simulink model "BLOC_Command"  (R2016a)
settings: Solver=VariableStepAuto  StartTime=0.0  StopTime=10.0  RelTol=1e-3
undefined symbols (not defined in the file): cmd_equivalent_conso_coef, cmd_qmax, cmd_specific_volume_l_per_g, fa_differential_ratio, fa_gearbox_efficiency, fa_gearbox_ratio, hev_dt, pla_wheel_radius, ra_differential_ratio, ra_transmission_efficiency
libraries: simulink x7
settings Model: Creator=Florent  LastModifiedBy=Florent
settings OptimizationCC: DefaultParameterBehavior=Inlined  OptimizeModelRefInitCode=on  LifeSpan=1
settings RTWCC: SystemTargetFile=ert.tlc  TemplateMakefile=ert_default_tmf  GenerateReport=on  IncludeHyperlinkInReport=on  LaunchReport=on  TargetLang=C++  GenerateTraceInfo=on  GenerateTraceReport=on  GenerateTraceReportSl=on  GenerateTraceReportSf=on  GenerateTraceReportEml=on
settings CodeAppCC: ForceParamTrailComments=on  OperatorAnnotations=on  SimulinkDataObjDesc=on  SFDataObjDesc=on  MATLABFcnDesc=on  InsertBlockDesc=on  MATLABSourceComments=on
settings ERTTargetCC: GenerateSampleERTMain=on  MultiInstanceERTCode=on  CodeInterfacePackaging=C++ class  InlinedParameterPlacement=NonHierarchical  RootIOFormat=Structure reference  ERTCustomFileTemplate=example_file_process.tlc

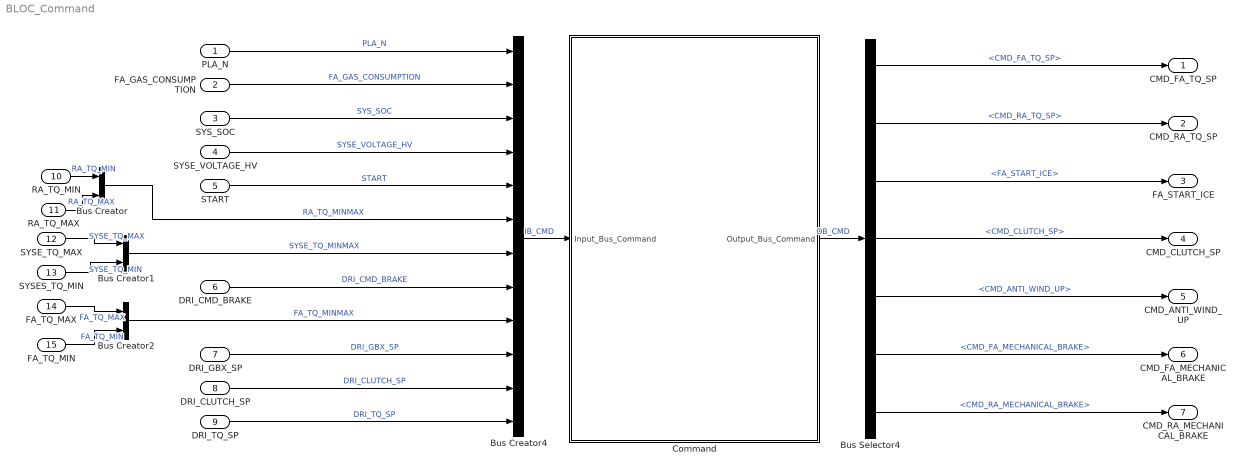
== system BLOC_Command ==
  PLA_N : Inport
  FA_GAS_CONSUMPTION : Inport  Port=2
  SYS_SOC : Inport  Port=3
  SYSE_VOLTAGE_HV : Inport  Port=4
  START : Inport  Port=5
  DRI_CMD_BRAKE : Inport  Port=6
  DRI_GBX_SP : Inport  Port=7
  DRI_CLUTCH_SP : Inport  Port=8
  DRI_TQ_SP : Inport  Port=9
  RA_TQ_MIN : Inport  Port=10
  RA_TQ_MAX : Inport  Port=11
  SYSE_TQ_MAX : Inport  Port=12
  SYSES_TQ_MIN : Inport  Port=13
  FA_TQ_MAX : Inport  Port=14
  FA_TQ_MIN : Inport  Port=15
  Bus Creator : BusCreator  Inputs=2
  Bus Creator1 : BusCreator  Inputs=2
  Bus Creator2 : BusCreator  Inputs=2
  Bus Creator4 : BusCreator  Inputs=12
  Bus Selector4 : BusSelector  OutputSignals=CMD_FA_TQ_SP,CMD_RA_TQ_SP,FA_START_ICE,CMD_CLUTCH_SP,CMD_ANTI_WIND_UP,CMD_FA_MECHANICAL_BRAKE,CMD_RA_MECHANICAL_BRAKE
  Command : Subsystem  TreatAsAtomicUnit=on
  CMD_FA_TQ_SP : Outport
  CMD_RA_TQ_SP : Outport  Port=2
  FA_START_ICE : Outport  Port=3
  CMD_CLUTCH_SP : Outport  Port=4
  CMD_ANTI_WIND_UP : Outport  Port=5
  CMD_FA_MECHANICAL_BRAKE : Outport  Port=6
  CMD_RA_MECHANICAL_BRAKE : Outport  Port=7
  wires:
  PLA_N/1 -> Bus Creator4/1  "PLA_N"
  FA_GAS_CONSUMPTION/1 -> Bus Creator4/2  "FA_GAS_CONSUMPTION"
  SYS_SOC/1 -> Bus Creator4/3  "SYS_SOC"
  SYSE_VOLTAGE_HV/1 -> Bus Creator4/4  "SYSE_VOLTAGE_HV"
  START/1 -> Bus Creator4/5  "START"
  Bus Creator/1 -> Bus Creator4/6  "RA_TQ_MINMAX"
  Bus Creator1/1 -> Bus Creator4/7  "SYSE_TQ_MINMAX"
  DRI_CMD_BRAKE/1 -> Bus Creator4/8  "DRI_CMD_BRAKE"
  Bus Creator2/1 -> Bus Creator4/9  "FA_TQ_MINMAX"
  DRI_GBX_SP/1 -> Bus Creator4/10  "DRI_GBX_SP"
  DRI_CLUTCH_SP/1 -> Bus Creator4/11  "DRI_CLUTCH_SP"
  DRI_TQ_SP/1 -> Bus Creator4/12  "DRI_TQ_SP"
  Bus Creator4/1 -> Command/1(Input_Bus_Command)  "IB_CMD"
  Command/1(Output_Bus_Command) -> Bus Selector4/1  "OB_CMD"
  Bus Selector4/1 -> CMD_FA_TQ_SP/1  "<CMD_FA_TQ_SP>"
  Bus Selector4/2 -> CMD_RA_TQ_SP/1  "<CMD_RA_TQ_SP>"
  Bus Selector4/3 -> FA_START_ICE/1  "<FA_START_ICE>"
  Bus Selector4/4 -> CMD_CLUTCH_SP/1  "<CMD_CLUTCH_SP>"
  Bus Selector4/5 -> CMD_ANTI_WIND_UP/1  "<CMD_ANTI_WIND_UP>"
  Bus Selector4/6 -> CMD_FA_MECHANICAL_BRAKE/1  "<CMD_FA_MECHANICAL_BRAKE>"
  Bus Selector4/7 -> CMD_RA_MECHANICAL_BRAKE/1  "<CMD_RA_MECHANICAL_BRAKE>"
  RA_TQ_MIN/1 -> Bus Creator/1  "RA_TQ_MIN"
  RA_TQ_MAX/1 -> Bus Creator/2  "RA_TQ_MAX"
  SYSE_TQ_MAX/1 -> Bus Creator1/1  "SYSE_TQ_MAX"
  SYSES_TQ_MIN/1 -> Bus Creator1/2  "SYSE_TQ_MIN"
  FA_TQ_MAX/1 -> Bus Creator2/1  "FA_TQ_MAX"
  FA_TQ_MIN/1 -> Bus Creator2/2  "FA_TQ_MIN"

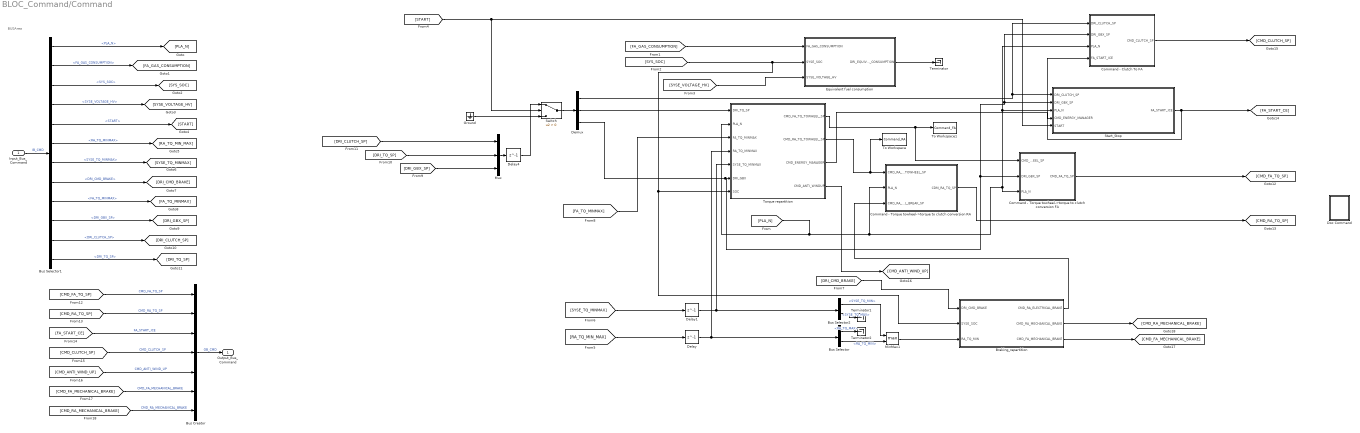
== system BLOC_Command/Command ==
  note: BUSArea
  Input_Bus_Command : Inport
  Braking_repartition : Subsystem
  Bus Creator : BusCreator  Inputs=7
  Bus Selector : BusSelector  OutputSignals=RA_TQ_MAX,RA_TQ_MIN
  Bus Selector1 : BusSelector  OutputSignals=PLA_N,FA_GAS_CONSUMPTION,SYS_SOC,SYSE_VOLTAGE_HV,START,RA_TQ_MINMAX,SYSE_TQ_MINMAX,DRI_CMD_BRAKE,FA_TQ_MINMAX,DRI_GBX_SP,DRI_CLUTCH_SP,DRI_TQ_SP
  Bus Selector2 : BusSelector  OutputSignals=SYSE_TQ_MIN,SYSE_TQ_MAX
  Command - Clutch To FA : Subsystem
  Command - Torque towheel->torque to clutch conversion FA : Subsystem
  Command - Torque towheel->torque to clutch conversion RA : Subsystem
  Delay : Delay  DelayLength=1
  Delay1 : Delay  DelayLength=1
  Delay4 : Delay  DelayLength=1  InitialCondition=1e-6
  Demux : Demux  Outputs=3
  Doc Command : Subsystem
      settings: OpenFcn=open('Documents\Command.pdf')
      mask Display: fprintf('DOC')
  Equivalent fuel consumption : Subsystem
  Ground : Ground
  MinMax1 : MinMax  Function=max  Inputs=2  SampleTime=hev_dt
  Mux : Mux  Inputs=3
  Start_Stop : Subsystem
  Switch : Switch  Criteria=u2 > Threshold
  Terminator : Terminator
  Terminator1 : Terminator
  Terminator2 : Terminator
  To Workspace : ToWorkspace  VariableName=Command_RA  SampleTime=-1
  To Workspace1 : ToWorkspace  VariableName=Command_FA  SampleTime=-1
  Torque repartition : Subsystem
  Output_Bus_Command : Outport
  wires:
  [FA_GAS_CONSUMPTION] -> Equivalent fuel consumption/1(FA_GAS_CONSUMPTION)
  [SYS_SOC] -> Equivalent fuel consumption/2(SYSE_SOC), Braking_repartition/2(SYSE_SOC), Torque repartition/7(SOC)
  [SYSE_VOLTAGE_HV] -> Equivalent fuel consumption/3(SYSE_VOLTAGE_HV)
  Torque repartition/1(CMD_FA_TQ_TOWHEEL_SP) -> To Workspace1/1, Command - Torque towheel->torque to clutch conversion FA/1(CMD_FA_TQ_TOWHEEL_SP)
  Equivalent fuel consumption/1(DRI_EQUIV_GAZ_CONSUMPTION) -> Terminator/1
  Command - Torque towheel->torque to clutch conversion FA/1(CMD_FA_TQ_SP) -> [CMD_FA_TQ_SP]
  [RA_TQ_MIN_MAX] -> Delay/1
  [SYSE_TQ_MINMAX] -> Delay1/1
  Bus Selector2/1 -> MinMax1/1  "<SYSE_TQ_MIN>"
  Bus Selector/2 -> MinMax1/2  "<RA_TQ_MIN>"
  Bus Selector/1 -> Terminator2/1  "<RA_TQ_MAX>"
  Bus Selector2/2 -> Terminator1/1  "<SYSE_TQ_MAX>"
  Command - Torque towheel->torque to clutch conversion RA/1(CDM_RA_TQ_SP) -> [CMD_RA_TQ_SP]
  Torque repartition/2(CMD_RA_TQ_TOWHEEL_SP) -> To Workspace/1, Command - Torque towheel->torque to clutch conversion RA/1(CMD_RA_TQ_TOWHEEL_SP)
  [START] -> Switch/2, Start_Stop/5(START)
  Start_Stop/1(FA_START_ICE) -> [FA_START_CE], Command - Clutch To FA/4(FA_START_ICE)
  [DRI_CMD_BRAKE] -> Braking_repartition/1(DRI_CMD_BRAKE)
  MinMax1/1 -> Braking_repartition/3(RA_TQ_MIN)
  [FA_TQ_MINMAX] -> Torque repartition/3(FA_TQ_MINMAX)
  Delay/1 -> Bus Selector/1, Torque repartition/4(RA_TQ_MINMAX)
  Delay1/1 -> Bus Selector2/1, Torque repartition/5(SYSE_TQ_MINMAX)
  Demux/1 -> Command - Clutch To FA/1(DRI_CLUTCH_SP), Start_Stop/1(DRI_CLUTCH_SP)
  [PLA_N] -> Command - Clutch To FA/3(PLA_N), Start_Stop/3(PLA_N), Command - Torque towheel->torque to clutch conversion FA/3(PLA_N), Command - Torque towheel->torque to clutch conversion RA/2(PLA_N), Torque repartition/2(PLA_N)
  Command - Clutch To FA/1("CMD_CLUTCH_SP ") -> [CMD_CLUTCH_SP]
  Torque repartition/3(CMD_ENERGY_MANAGER) -> Start_Stop/4(CMD_ENERGY_MANAGER)
  Torque repartition/4(CMD_ANTI_WINDUP) -> [CMD_ANTI_WIND_UP]
  Switch/1 -> Demux/1
  [DRI_GBX_SP] -> Mux/3
  Mux/1 -> Delay4/1
  Demux/3 -> Command - Clutch To FA/2(DRI_GBX_SP), Start_Stop/2(DRI_GBX_SP), Command - Torque towheel->torque to clutch conversion FA/2(DRI_GBX_SP), Torque repartition/6(DRI_GBX)
  Delay4/1 -> Switch/1
  Ground/1 -> Switch/3
  [DRI_CLUTCH_SP] -> Mux/1
  [DRI_TQ_SP] -> Mux/2
  Demux/2 -> Torque repartition/1(DRI_TQ_SP)
  Braking_repartition/1(CMD_RA_ELECTRICAL_BRAKE) -> Command - Torque towheel->torque to clutch conversion RA/3(CMD_RA_TQ_TOWHEEL_BREAK_SP)
  Braking_repartition/3(CMD_FA_MECHANICAL_BRAKE) -> [CMD_FA_MECHANICAL_BRAKE]
  Braking_repartition/2(CMD_RA_MECHANICAL_BRAKE) -> [CMD_RA_MECHANICAL_BRAKE]
  Input_Bus_Command/1 -> Bus Selector1/1  "IB_CMD"
  Bus Selector1/1 -> [PLA_N]  "<PLA_N>"
  Bus Selector1/2 -> [FA_GAS_CONSUMPTION]  "<FA_GAS_CONSUMPTION>"
  Bus Selector1/3 -> [SYS_SOC]  "<SYS_SOC>"
  Bus Selector1/4 -> [SYSE_VOLTAGE_HV]  "<SYSE_VOLTAGE_HV>"
  Bus Selector1/5 -> [START]  "<START>"
  Bus Selector1/6 -> [RA_TQ_MIN_MAX]  "<RA_TQ_MINMAX>"
  Bus Selector1/7 -> [SYSE_TQ_MINMAX]  "<SYSE_TQ_MINMAX>"
  Bus Selector1/8 -> [DRI_CMD_BRAKE]  "<DRI_CMD_BRAKE>"
  Bus Selector1/9 -> [FA_TQ_MINMAX]  "<FA_TQ_MINMAX>"
  Bus Selector1/10 -> [DRI_GBX_SP]  "<DRI_GBX_SP>"
  Bus Selector1/11 -> [DRI_CLUTCH_SP]  "<DRI_CLUTCH_SP>"
  Bus Selector1/12 -> [DRI_TQ_SP]  "<DRI_TQ_SP>"
  Bus Creator/1 -> Output_Bus_Command/1  "OB_CMD"
  [CMD_FA_TQ_SP] -> Bus Creator/1  "CMD_FA_TQ_SP"
  [CMD_RA_TQ_SP] -> Bus Creator/2  "CMD_RA_TQ_SP"
  [FA_START_CE] -> Bus Creator/3  "FA_START_ICE"
  [CMD_CLUTCH_SP] -> Bus Creator/4  "CMD_CLUTCH_SP"
  [CMD_ANTI_WIND_UP] -> Bus Creator/5  "CMD_ANTI_WIND_UP"
  [CMD_FA_MECHANICAL_BRAKE] -> Bus Creator/6  "CMD_FA_MECHANICAL_BRAKE"
  [CMD_RA_MECHANICAL_BRAKE] -> Bus Creator/7  "CMD_RA_MECHANICAL_BRAKE"

== system BLOC_Command/Command/Braking_repartition ==
  DRI_CMD_BRAKE : Inport
  SYSE_SOC : Inport  Port=2
  RA_TQ_MIN : Inport  Port=3
  BREAK REPARTITION FRONT/REAR : Subsystem
  BREAKE REPARTITION RA : Subsystem
  CMD_RA_ELECTRICAL_BRAKE : Outport
  CMD_RA_MECHANICAL_BRAKE : Outport  Port=2
  CMD_FA_MECHANICAL_BRAKE : Outport  Port=3
  wires:
  DRI_CMD_BRAKE/1 -> BREAK REPARTITION FRONT/REAR/1(DRI_CMD_BRAKE)
  BREAK REPARTITION FRONT/REAR/1(CMD_FA_BRAKE) -> CMD_FA_MECHANICAL_BRAKE/1
  BREAK REPARTITION FRONT/REAR/2(CMD_RA_BRAKE) -> BREAKE REPARTITION RA/1(CMD_RA_BREAK)
  SYSE_SOC/1 -> BREAKE REPARTITION RA/2(SYSE_SOC)
  RA_TQ_MIN/1 -> BREAKE REPARTITION RA/3(RA_TQ_MIN)
  BREAKE REPARTITION RA/1(CMD_RA_MECHANICAL_BRAKE) -> CMD_RA_MECHANICAL_BRAKE/1
  BREAKE REPARTITION RA/2(CMD_RA_ELECTRICAL_BRAKE) -> CMD_RA_ELECTRICAL_BRAKE/1

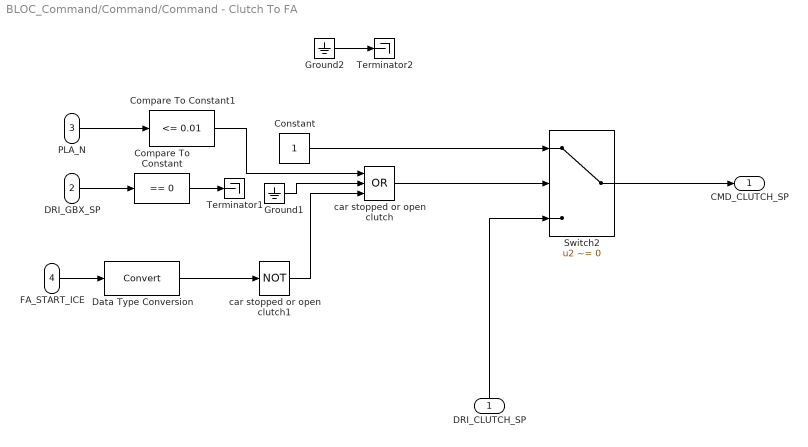
== system BLOC_Command/Command/Command - Clutch To FA ==
  DRI_CLUTCH_SP : Inport
  DRI_GBX_SP : Inport  Port=2
  PLA_N : Inport  Port=3
  FA_START_ICE : Inport  Port=4
  Compare To Constant : simulink/Logic and Bit Operations/Compare To Constant  relop===  const=0  OutDataTypeStr=uint8
  Compare To Constant1 : simulink/Logic and Bit Operations/Compare To Constant  relop=<=  const=0.01  OutDataTypeStr=uint8
  Constant : Constant
  Data Type Conversion : DataTypeConversion
  Ground1 : Ground
  Ground2 : Ground
  Switch2 : Switch  Criteria=u2 ~= 0  Threshold=1
  Terminator1 : Terminator
  Terminator2 : Terminator
  car stopped or open clutch : Logic  Operator=OR  Inputs=3  AllPortsSameDT=off  OutDataTypeStr=boolean
  car stopped or open clutch1 : Logic  Operator=NOT  Inputs=3  AllPortsSameDT=off  OutDataTypeStr=boolean
  "CMD_CLUTCH_SP " : Outport
  wires:
  Switch2/1 -> "CMD_CLUTCH_SP "/1
  DRI_GBX_SP/1 -> Compare To Constant/1
  Compare To Constant/1 -> Terminator1/1
  car stopped or open clutch/1 -> Switch2/2
  DRI_CLUTCH_SP/1 -> Switch2/3
  PLA_N/1 -> Compare To Constant1/1
  Constant/1 -> Switch2/1
  FA_START_ICE/1 -> Data Type Conversion/1
  Data Type Conversion/1 -> car stopped or open clutch1/1
  Compare To Constant1/1 -> car stopped or open clutch/1
  Ground1/1 -> car stopped or open clutch/2
  car stopped or open clutch1/1 -> car stopped or open clutch/3
  Ground2/1 -> Terminator2/1

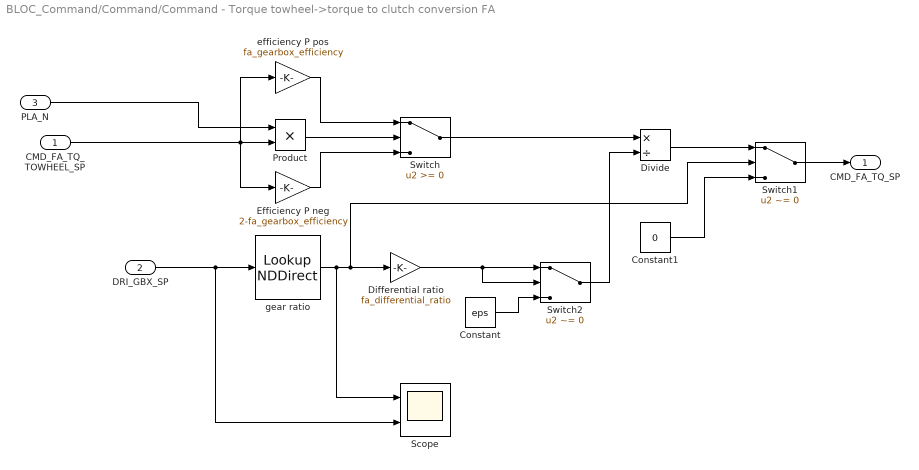
== system BLOC_Command/Command/Command - Torque towheel->torque to clutch conversion FA ==
  CMD_FA_TQ_TOWHEEL_SP : Inport
  DRI_GBX_SP : Inport  Port=2
  PLA_N : Inport  Port=3
  Constant : Constant  Value=eps
  Constant1 : Constant  Value=0
  Differential ratio : Gain  Gain=fa_differential_ratio  SampleTime=hev_dt
  Divide : Product  Inputs=*/
  Efficiency P neg : Gain  Gain=2-fa_gearbox_efficiency  SampleTime=hev_dt
  Product : Product  SampleTime=hev_dt
  Scope : Scope  NumInputPorts=2
  Switch : Switch  SampleTime=hev_dt
  Switch1 : Switch  Criteria=u2 ~= 0  SampleTime=hev_dt
  Switch2 : Switch  Criteria=u2 ~= 0  SampleTime=hev_dt
  efficiency P pos : Gain  Gain=fa_gearbox_efficiency  SampleTime=hev_dt
  gear ratio : LookupNDDirect  NumberOfTableDimensions=1  Table=fa_gearbox_ratio  SampleTime=hev_dt
  CMD_FA_TQ_SP : Outport
  wires:
  DRI_GBX_SP/1 -> Scope/2, gear ratio/1
  gear ratio/1 -> Scope/1, Switch1/2, Differential ratio/1
  CMD_FA_TQ_TOWHEEL_SP/1 -> Product/2, Efficiency P neg/1, efficiency P pos/1
  efficiency P pos/1 -> Switch/1
  Efficiency P neg/1 -> Switch/3
  Product/1 -> Switch/2
  Switch/1 -> Divide/1
  PLA_N/1 -> Product/1
  Constant1/1 -> Switch1/3
  Switch1/1 -> CMD_FA_TQ_SP/1
  Divide/1 -> Switch1/1
  Constant/1 -> Switch2/3
  Switch2/1 -> Divide/2
  Differential ratio/1 -> Switch2/2, Switch2/1

== system BLOC_Command/Command/Command - Torque towheel->torque to clutch conversion RA ==
  CMD_RA_TQ_TOWHEEL_SP : Inport
  PLA_N : Inport  Port=2
  CMD_RA_TQ_TOWHEEL_BREAK_SP : Inport  Port=3
  Differential ratio : Gain  Gain=1/ra_differential_ratio  SampleTime=hev_dt
  Efficiency P neg : Gain  Gain=2-ra_transmission_efficiency  SampleTime=hev_dt
  Efficiency P pos : Gain  Gain=ra_transmission_efficiency  SampleTime=hev_dt
  Product : Product  SampleTime=hev_dt
  Sum : Sum  Inputs=|+-
  Switch : Switch  SampleTime=hev_dt
  CDM_RA_TQ_SP : Outport
  wires:
  CMD_RA_TQ_TOWHEEL_SP/1 -> Sum/1
  Efficiency P pos/1 -> Switch/1
  Efficiency P neg/1 -> Switch/3
  Product/1 -> Switch/2
  PLA_N/1 -> Product/1
  Differential ratio/1 -> CDM_RA_TQ_SP/1
  Switch/1 -> Differential ratio/1
  Sum/1 -> Product/2, Efficiency P pos/1, Efficiency P neg/1
  CMD_RA_TQ_TOWHEEL_BREAK_SP/1 -> Sum/2

== system BLOC_Command/Command/Doc Command ==

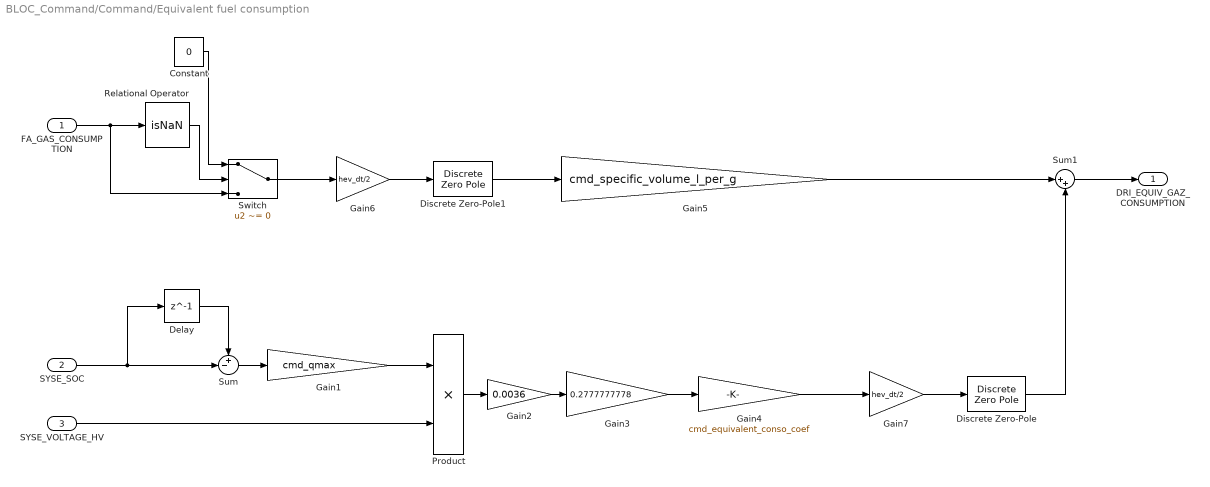
== system BLOC_Command/Command/Equivalent fuel consumption ==
  FA_GAS_CONSUMPTION : Inport
  SYSE_SOC : Inport  Port=2
  SYSE_VOLTAGE_HV : Inport  Port=3
  Constant : Constant  Value=0
  Delay : Delay  DelayLength=1  SampleTime=hev_dt
  Discrete Zero-Pole : DiscreteZeroPole  Zeros=[-1]  Poles=[1]  Gain=1  SampleTime=hev_dt
  Discrete Zero-Pole1 : DiscreteZeroPole  Zeros=[-1]  Poles=[1]  Gain=1  SampleTime=hev_dt
  Gain1 : Gain  Gain=cmd_qmax  SampleTime=hev_dt
  Gain2 : Gain  Gain=0.0036  SampleTime=hev_dt
  Gain3 : Gain  Gain=0.2777777778  SampleTime=hev_dt
  Gain4 : Gain  Gain=cmd_equivalent_conso_coef  SampleTime=hev_dt
  Gain5 : Gain  Gain=cmd_specific_volume_l_per_g  SampleTime=hev_dt
  Gain6 : Gain  Gain=hev_dt/2  SampleTime=hev_dt
  Gain7 : Gain  Gain=hev_dt/2  SampleTime=hev_dt
  Product : Product  SampleTime=hev_dt
  Relational Operator : RelationalOperator  Operator=isNaN  OutDataTypeStr=boolean  SampleTime=hev_dt
  Sum : Sum  Inputs=+-|  SampleTime=hev_dt
  Sum1 : Sum  Inputs=|++  SampleTime=hev_dt
  Switch : Switch  Criteria=u2 ~= 0  SampleTime=hev_dt
  DRI_EQUIV_GAZ_CONSUMPTION : Outport
  wires:
  Gain2/1 -> Gain3/1
  Product/1 -> Gain2/1
  SYSE_SOC/1 -> Delay/1, Sum/2
  Delay/1 -> Sum/1
  Sum/1 -> Gain1/1
  SYSE_VOLTAGE_HV/1 -> Product/2
  Gain3/1 -> Gain4/1
  Sum1/1 -> DRI_EQUIV_GAZ_CONSUMPTION/1
  Gain5/1 -> Sum1/1
  Discrete Zero-Pole/1 -> Sum1/2
  Gain1/1 -> Product/1
  FA_GAS_CONSUMPTION/1 -> Relational Operator/1, Switch/3
  Relational Operator/1 -> Switch/2
  Constant/1 -> Switch/1
  Gain4/1 -> Gain7/1
  Gain7/1 -> Discrete Zero-Pole/1
  Switch/1 -> Gain6/1
  Discrete Zero-Pole1/1 -> Gain5/1
  Gain6/1 -> Discrete Zero-Pole1/1

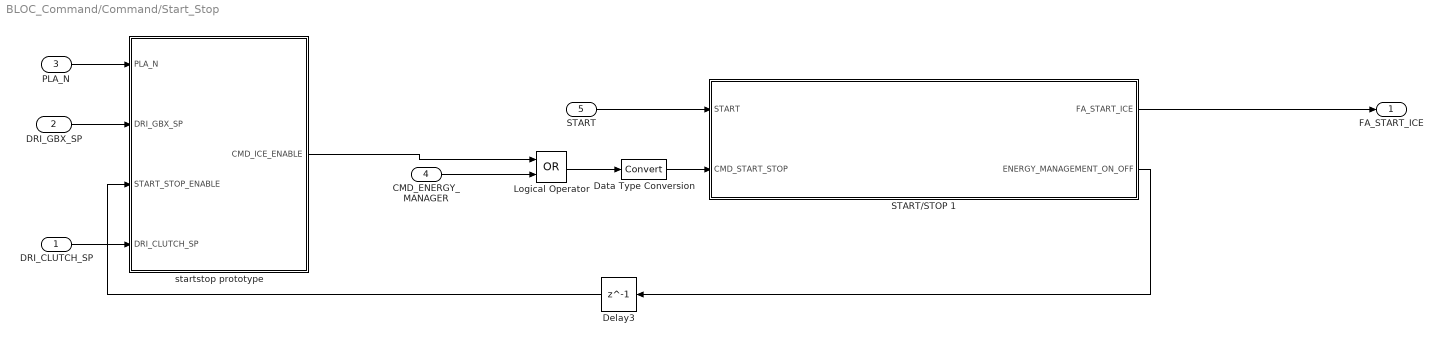
== system BLOC_Command/Command/Start_Stop ==
  DRI_CLUTCH_SP : Inport
  DRI_GBX_SP : Inport  Port=2
  PLA_N : Inport  Port=3
  CMD_ENERGY_MANAGER : Inport  Port=4
  START : Inport  Port=5
  Data Type Conversion : DataTypeConversion
  Delay3 : Delay  DelayLength=1
  Logical Operator : Logic  Operator=OR  AllPortsSameDT=off  OutDataTypeStr=boolean
  START/STOP 1 : Stateflow chart  TreatAsAtomicUnit=on
  startstop prototype : Subsystem
  FA_START_ICE : Outport
  wires:
  DRI_CLUTCH_SP/1 -> startstop prototype/4(DRI_CLUTCH_SP)
  PLA_N/1 -> startstop prototype/1(PLA_N)
  DRI_GBX_SP/1 -> startstop prototype/2(DRI_GBX_SP)
  START/STOP 1/2(ENERGY_MANAGEMENT_ON_OFF) -> Delay3/1
  startstop prototype/1(CMD_ICE_ENABLE) -> Logical Operator/1
  CMD_ENERGY_MANAGER/1 -> Logical Operator/2
  Logical Operator/1 -> Data Type Conversion/1
  START/1 -> START/STOP 1/1(START)
  Delay3/1 -> startstop prototype/3(START_STOP_ENABLE)
  Data Type Conversion/1 -> START/STOP 1/2(CMD_START_STOP)
  START/STOP 1/1(FA_START_ICE) -> FA_START_ICE/1

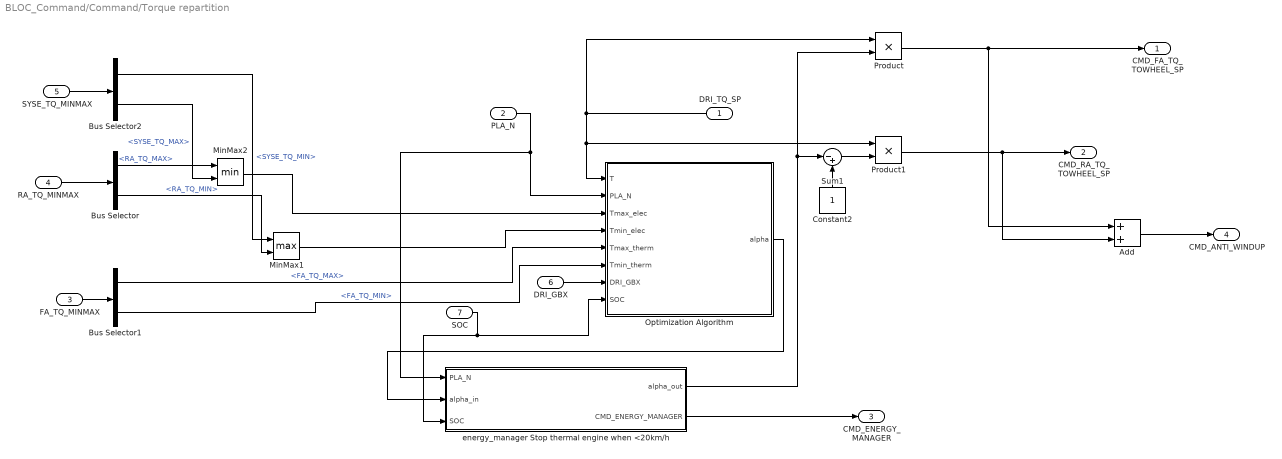
== system BLOC_Command/Command/Torque repartition ==
  DRI_TQ_SP : Inport
  PLA_N : Inport  Port=2
  FA_TQ_MINMAX : Inport  Port=3
  RA_TQ_MINMAX : Inport  Port=4
  SYSE_TQ_MINMAX : Inport  Port=5
  DRI_GBX : Inport  Port=6
  SOC : Inport  Port=7
  Add : Sum
  Bus Selector : BusSelector  OutputSignals=RA_TQ_MAX,RA_TQ_MIN
  Bus Selector1 : BusSelector  OutputSignals=FA_TQ_MAX,FA_TQ_MIN
  Bus Selector2 : BusSelector  OutputSignals=SYSE_TQ_MIN,SYSE_TQ_MAX
  Constant2 : Constant
  MinMax1 : MinMax  Function=max  Inputs=2  SampleTime=hev_dt
  MinMax2 : MinMax  Inputs=2  SampleTime=hev_dt
  "Optimization Algorithm " : Subsystem
  Product : Product
  Product1 : Product
  Sum1 : Sum  Inputs=|-+
  energy_manager Stop thermal engine when <20km/h : Subsystem
  CMD_FA_TQ_TOWHEEL_SP : Outport
  CMD_RA_TQ_TOWHEEL_SP : Outport  Port=2
  CMD_ENERGY_MANAGER : Outport  Port=3
  CMD_ANTI_WINDUP : Outport  Port=4
  wires:
  Product1/1 -> Add/2, CMD_RA_TQ_TOWHEEL_SP/1
  PLA_N/1 -> "Optimization Algorithm "/2(PLA_N), energy_manager Stop thermal engine when <20km/h/1(PLA_N)
  Sum1/1 -> Product1/2
  MinMax2/1 -> "Optimization Algorithm "/3(Tmax_elec)
  MinMax1/1 -> "Optimization Algorithm "/4(Tmin_elec)
  Constant2/1 -> Sum1/2
  RA_TQ_MINMAX/1 -> Bus Selector/1
  SYSE_TQ_MINMAX/1 -> Bus Selector2/1
  Bus Selector2/1 -> MinMax1/1  "<SYSE_TQ_MIN>"
  Bus Selector/2 -> MinMax1/2  "<RA_TQ_MIN>"
  Bus Selector/1 -> MinMax2/1  "<RA_TQ_MAX>"
  Bus Selector2/2 -> MinMax2/2  "<SYSE_TQ_MAX>"
  FA_TQ_MINMAX/1 -> Bus Selector1/1
  DRI_GBX/1 -> "Optimization Algorithm "/7(DRI_GBX)
  Bus Selector1/1 -> "Optimization Algorithm "/5(Tmax_therm)  "<FA_TQ_MAX>"
  Bus Selector1/2 -> "Optimization Algorithm "/6(Tmin_therm)  "<FA_TQ_MIN>"
  DRI_TQ_SP/1 -> Product1/1, "Optimization Algorithm "/1(T), Product/1
  SOC/1 -> "Optimization Algorithm "/8("SOC "), energy_manager Stop thermal engine when <20km/h/3(SOC)
  energy_manager Stop thermal engine when <20km/h/1(alpha_out) -> Product/2, Sum1/1
  "Optimization Algorithm "/1(alpha) -> energy_manager Stop thermal engine when <20km/h/2(alpha_in)
  energy_manager Stop thermal engine when <20km/h/2(CMD_ENERGY_MANAGER) -> CMD_ENERGY_MANAGER/1
  Product/1 -> Add/1, CMD_FA_TQ_TOWHEEL_SP/1
  Add/1 -> CMD_ANTI_WINDUP/1

== system BLOC_Command/Command/Braking_repartition/BREAK REPARTITION FRONT//REAR ==
  DRI_CMD_BRAKE : Inport
  Gain : Gain  Gain=2/3
  Gain1 : Gain  Gain=1/3
  CMD_FA_BRAKE : Outport
  CMD_RA_BRAKE : Outport  Port=2
  wires:
  Gain/1 -> CMD_FA_BRAKE/1
  Gain1/1 -> CMD_RA_BRAKE/1
  DRI_CMD_BRAKE/1 -> Gain1/1, Gain/1

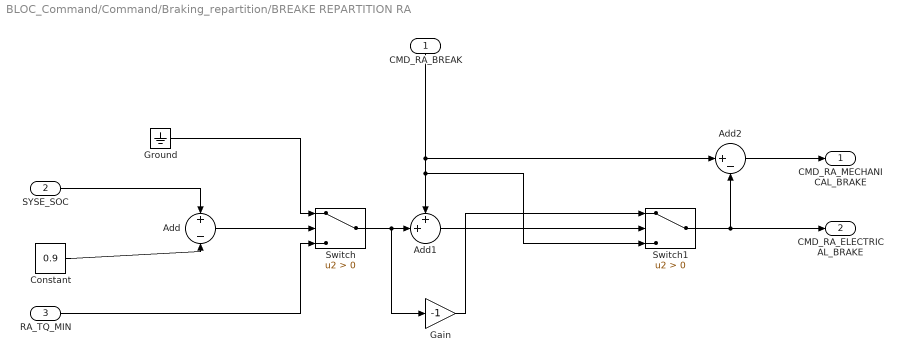
== system BLOC_Command/Command/Braking_repartition/BREAKE REPARTITION RA ==
  CMD_RA_BREAK : Inport
  SYSE_SOC : Inport  Port=2
  RA_TQ_MIN : Inport  Port=3
  Add : Sum  Inputs=+-
  Add1 : Sum  Inputs=++|
  Add2 : Sum  Inputs=|+-
  Constant : Constant  Tag=Soc_level  Value=0.9
  Gain : Gain  Gain=-1
  Ground : Ground
  Switch : Switch  Criteria=u2 > Threshold
  Switch1 : Switch  Criteria=u2 > Threshold
  CMD_RA_MECHANICAL_BRAKE : Outport
  CMD_RA_ELECTRICAL_BRAKE : Outport  Port=2
  wires:
  CMD_RA_BREAK/1 -> Add1/1, Switch1/3, Add2/1
  Switch1/1 -> CMD_RA_ELECTRICAL_BRAKE/1, Add2/2
  Add1/1 -> Switch1/2
  Ground/1 -> Switch/1
  RA_TQ_MIN/1 -> Switch/3
  Switch/1 -> Gain/1, Add1/2
  Add2/1 -> CMD_RA_MECHANICAL_BRAKE/1
  SYSE_SOC/1 -> Add/1
  Constant/1 -> Add/2
  Add/1 -> Switch/2
  Gain/1 -> Switch1/1

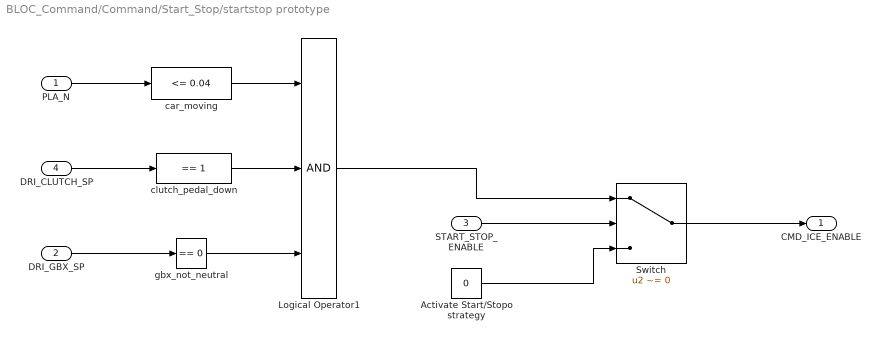
== system BLOC_Command/Command/Start_Stop/startstop prototype ==
  PLA_N : Inport
  DRI_GBX_SP : Inport  Port=2
  START_STOP_ENABLE : Inport  Port=3
  DRI_CLUTCH_SP : Inport  Port=4
  Activate Start/Stopo strategy : Constant  Value=0
  Logical Operator1 : Logic  Inputs=3  AllPortsSameDT=off  OutDataTypeStr=boolean  SampleTime=hev_dt
  Switch : Switch  Criteria=u2 ~= 0  SampleTime=hev_dt
  car_moving : simulink/Logic and Bit Operations/Compare To Constant  relop=<=  const=0.04  OutDataTypeStr=uint8
  clutch_pedal_down : simulink/Logic and Bit Operations/Compare To Constant  relop===  const=1  OutDataTypeStr=uint8
  gbx_not_neutral : simulink/Logic and Bit Operations/Compare To Constant  relop===  const=0  OutDataTypeStr=uint8
  CMD_ICE_ENABLE : Outport
  wires:
  PLA_N/1 -> car_moving/1
  car_moving/1 -> Logical Operator1/1
  gbx_not_neutral/1 -> Logical Operator1/3
  Activate Start/Stopo strategy/1 -> Switch/3
  Logical Operator1/1 -> Switch/1
  DRI_GBX_SP/1 -> gbx_not_neutral/1
  START_STOP_ENABLE/1 -> Switch/2
  Switch/1 -> CMD_ICE_ENABLE/1
  DRI_CLUTCH_SP/1 -> clutch_pedal_down/1
  clutch_pedal_down/1 -> Logical Operator1/2

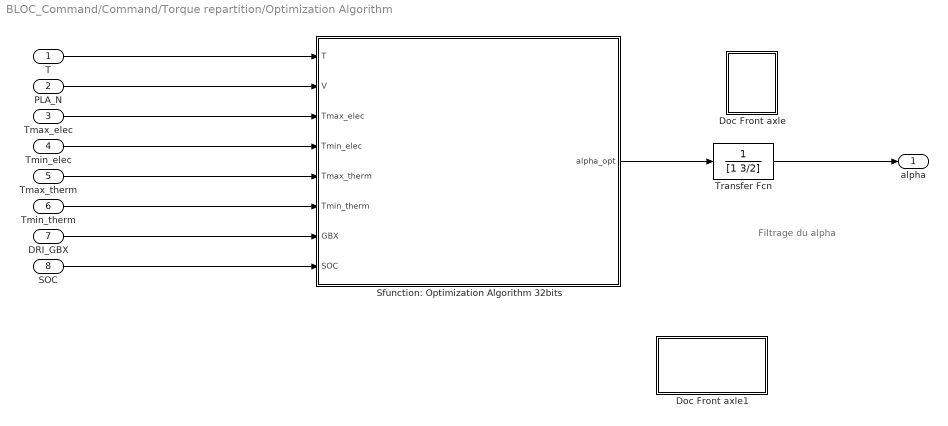
== system BLOC_Command/Command/Torque repartition/Optimization Algorithm  ==
  note: Filtrage du alpha
  T : Inport
  PLA_N : Inport  Port=2
  Tmax_elec : Inport  Port=3
  Tmin_elec : Inport  Port=4
  Tmax_therm : Inport  Port=5
  Tmin_therm : Inport  Port=6
  DRI_GBX : Inport  Port=7
  "SOC " : Inport  Port=8
  Doc Front axle : Subsystem
      settings: OpenFcn=open('Documents\Command Torque Repartition Algorithm.pdf')
      mask Display: fprintf('DOC')
  Doc Front axle1 : Subsystem
      settings: OpenFcn=open('Optimization_Algorithm')
      mask Display: fprintf('Generate\nOptimization\nAlgorithm\nSfunction')
  Sfunction: Optimization Algorithm 32bits : Subsystem
      mask help: Simulink:masks:GenSFuncDesc_MD
      mask Help: eval('feval(''rtwprivate'',''rtwhelpview'',''rtw_sfcn_block'')');
  Transfer Fcn : TransferFcn  Denominator=[1 3/2]
  alpha : Outport
  wires:
  Tmax_elec/1 -> Sfunction: Optimization Algorithm 32bits/3(Tmax_elec)
  Tmin_elec/1 -> Sfunction: Optimization Algorithm 32bits/4(Tmin_elec)
  PLA_N/1 -> Sfunction: Optimization Algorithm 32bits/2(V)
  Tmax_therm/1 -> Sfunction: Optimization Algorithm 32bits/5(Tmax_therm)
  T/1 -> Sfunction: Optimization Algorithm 32bits/1(T)
  Tmin_therm/1 -> Sfunction: Optimization Algorithm 32bits/6(Tmin_therm)
  DRI_GBX/1 -> Sfunction: Optimization Algorithm 32bits/7(GBX)
  "SOC "/1 -> Sfunction: Optimization Algorithm 32bits/8(SOC)
  Transfer Fcn/1 -> alpha/1
  Sfunction: Optimization Algorithm 32bits/1(alpha_opt) -> Transfer Fcn/1

== system BLOC_Command/Command/Torque repartition/energy_manager Stop thermal engine when <20km//h ==
  note: Energy managment modified : Not taking account of the FA_START command
      | Cf. Previous model
  PLA_N : Inport
  alpha_in : Inport  Port=2
  SOC : Inport  Port=3
  Compare To Constant : simulink/Logic and Bit Operations/Compare To Constant  relop=<  const=20  OutDataTypeStr=boolean
  Compare To Constant1 : simulink/Logic and Bit Operations/Compare To Constant  relop=>  const=0.2  OutDataTypeStr=boolean
  Constant3 : Constant  Value=0
  Gain : Gain  Gain=(60*(2*pi*pla_wheel_radius))/1e3
  Logical Operator1 : Logic  AllPortsSameDT=off  OutDataTypeStr=boolean
  Switch : Switch  Criteria=u2 > Threshold
  alpha_out : Outport
  CMD_ENERGY_MANAGER : Outport  Port=2
  wires:
  SOC/1 -> Compare To Constant1/1
  PLA_N/1 -> Gain/1
  Logical Operator1/1 -> CMD_ENERGY_MANAGER/1, Switch/2
  Compare To Constant1/1 -> Logical Operator1/1
  Gain/1 -> Compare To Constant/1
  Constant3/1 -> Switch/1
  alpha_in/1 -> Switch/3
  Switch/1 -> alpha_out/1
  Compare To Constant/1 -> Logical Operator1/2

== system BLOC_Command/Command/Torque repartition/Optimization Algorithm /Doc Front axle ==

== system BLOC_Command/Command/Torque repartition/Optimization Algorithm /Doc Front axle1 ==

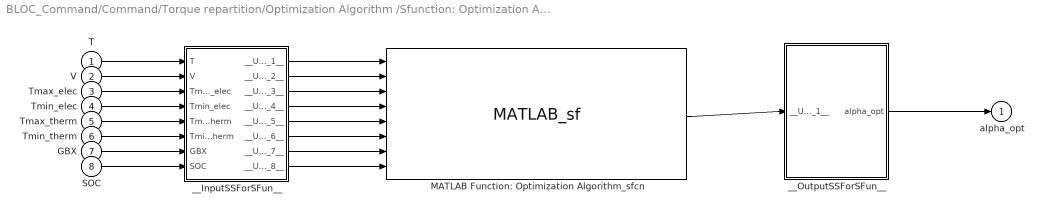
== system BLOC_Command/Command/Torque repartition/Optimization Algorithm /Sfunction: Optimization Algorithm 32bits ==
  T : Inport
  V : Inport  Port=2
  Tmax_elec : Inport  Port=3
  Tmin_elec : Inport  Port=4
  Tmax_therm : Inport  Port=5
  Tmin_therm : Inport  Port=6
  GBX : Inport  Port=7
  SOC : Inport  Port=8
  MATLAB Function: Optimization Algorithm_sfcn : S-Function  FunctionName=MATLAB_sf  SFunctionModules=""  SFunctionDeploymentMode=off  EnableBusSupport=off  mask{rtw_sf_name=MATLAB_sf, showVar=off}
      mask prompts: rtw_sf_name "Simulink:masks:GenSFuncName_MP"; showVar "Simulink:masks:GenSFuncShowModuleList_MP"
      mask help: Simulink:masks:GenSFuncDesc_MD
      mask init:
      | displist = '';
      | if ~strcmp(get_param(gcb, 'FunctionName'), rtw_sf_name);
      |   set_param(gcb, 'FunctionName', rtw_sf_name);
      | end
      | % Check if we are generating code
      | rtw_mode = false;
      | if strcmpi(get_param(bdroot(gcb),'SimulationStatus'),'Initializing')
      | 	rtw_mode = strcmpi(get_param(bdroot(gcb),'BuildingRTWCode'),'on') && ...
      | 		~strcmpi(get_param(bdroot(gcb),'TargetStyle'),'SimulationTarget');
      | end
      | if showVar || rtw_mode
      | 	if exist('rtwsfunc') == 2 | exist('rtwsfunc') == 6
      | 		tmplist = rtwsfunc(rtw_sf_name,gcb);
      | 		tmplist = DAStudio.message('Simulink:masks:GenSFuncListOfModules_IC', tmplist);
      | 	elseif showVar
      | 		tmplist1 = DAStudio.message('Simulink:masks:GenSFuncListOfModules_IC', '');
      |         tmplist2 = DAStudio.message('Simulink:masks:GenSFuncNotLicensed_IC');
      |         tmplist = [tmplist1 tmplist2];
      |  	end
      | end
      | if showVar
      |   displist = tmplist;
      | end
      settings: CopyFcn=|
      | if ~strcmp(get_param(gcb,'Linkstatus'),'none') && ...
      | ~strcmp(get_param(gcb,'Linkstatus'),'implicit')
      |   set_param(gcb,'LinkStatus','none');
      | end
      mask Help: eval('feval(''rtwprivate'',''rtwhelpview'',''rtw_sfcn_block'')');
      mask Display:
      | port_label('input',1,'T');
      | port_label('input',2,'V');
      | port_label('input',3,'Tmax_elec');
      | port_label('input',4,'Tmin_elec');
      | port_label('input',5,'Tmax_therm');
      | port_label('input',6,'Tmin_therm');
      | port_label('input',7,'GBX');
      | port_label('input',8,'SOC');
      | port_label('output',1,'alpha_opt');
  __InputSSForSFun__ : Subsystem
  __OutputSSForSFun__ : Subsystem
  alpha_opt : Outport
  wires:
  T/1 -> __InputSSForSFun__/1(T)
  V/1 -> __InputSSForSFun__/2(V)
  Tmax_elec/1 -> __InputSSForSFun__/3(Tmax_elec)
  Tmin_elec/1 -> __InputSSForSFun__/4(Tmin_elec)
  Tmax_therm/1 -> __InputSSForSFun__/5(Tmax_therm)
  Tmin_therm/1 -> __InputSSForSFun__/6(Tmin_therm)
  GBX/1 -> __InputSSForSFun__/7(GBX)
  SOC/1 -> __InputSSForSFun__/8(SOC)
  __InputSSForSFun__/1(__UniqueOutportName__1__) -> MATLAB Function: Optimization Algorithm_sfcn/1
  __InputSSForSFun__/2(__UniqueOutportName__2__) -> MATLAB Function: Optimization Algorithm_sfcn/2
  __InputSSForSFun__/3(__UniqueOutportName__3__) -> MATLAB Function: Optimization Algorithm_sfcn/3
  __InputSSForSFun__/4(__UniqueOutportName__4__) -> MATLAB Function: Optimization Algorithm_sfcn/4
  __InputSSForSFun__/5(__UniqueOutportName__5__) -> MATLAB Function: Optimization Algorithm_sfcn/5
  __InputSSForSFun__/6(__UniqueOutportName__6__) -> MATLAB Function: Optimization Algorithm_sfcn/6
  __InputSSForSFun__/7(__UniqueOutportName__7__) -> MATLAB Function: Optimization Algorithm_sfcn/7
  __InputSSForSFun__/8(__UniqueOutportName__8__) -> MATLAB Function: Optimization Algorithm_sfcn/8
  MATLAB Function: Optimization Algorithm_sfcn/1 -> __OutputSSForSFun__/1(__UniqueInportName__1__)
  __OutputSSForSFun__/1(alpha_opt) -> alpha_opt/1

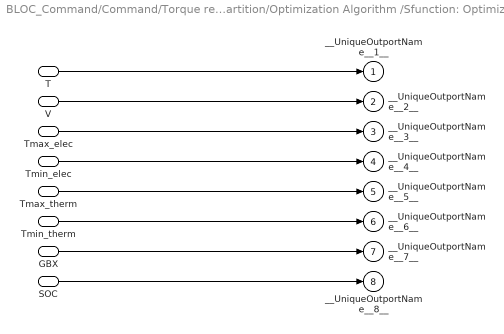
== system BLOC_Command/Command/Torque repartition/Optimization Algorithm /Sfunction: Optimization Algorithm 32bits/__InputSSForSFun__ ==
  T : Inport
  V : Inport  Port=2
  Tmax_elec : Inport  Port=3
  Tmin_elec : Inport  Port=4
  Tmax_therm : Inport  Port=5
  Tmin_therm : Inport  Port=6
  GBX : Inport  Port=7
  SOC : Inport  Port=8
  __UniqueOutportName__1__ : Outport
  __UniqueOutportName__2__ : Outport  Port=2
  __UniqueOutportName__3__ : Outport  Port=3
  __UniqueOutportName__4__ : Outport  Port=4
  __UniqueOutportName__5__ : Outport  Port=5
  __UniqueOutportName__6__ : Outport  Port=6
  __UniqueOutportName__7__ : Outport  Port=7
  __UniqueOutportName__8__ : Outport  Port=8
  wires:
  T/1 -> __UniqueOutportName__1__/1
  V/1 -> __UniqueOutportName__2__/1
  Tmax_elec/1 -> __UniqueOutportName__3__/1
  Tmin_elec/1 -> __UniqueOutportName__4__/1
  Tmax_therm/1 -> __UniqueOutportName__5__/1
  Tmin_therm/1 -> __UniqueOutportName__6__/1
  GBX/1 -> __UniqueOutportName__7__/1
  SOC/1 -> __UniqueOutportName__8__/1

== system BLOC_Command/Command/Torque repartition/Optimization Algorithm /Sfunction: Optimization Algorithm 32bits/__OutputSSForSFun__ ==
  __UniqueInportName__1__ : Inport
  alpha_opt : Outport
  wires:
  __UniqueInportName__1__/1 -> alpha_opt/1  "alpha_opt"

== stateflow chart BLOC_Command/Command/Start_Stop/START//STOP 1 ==
  state WAKEUP
    entry:ENERGY_MANAGEMENT_ON_OFF=0;
  state RUNNING
    entry: ENERGY_MANAGEMENT_ON_OFF=1;
    entry: FA_START_ICE=0;
    state START
      entry: FA_START_ICE=1;
      k = 0;
      during : k = k+1;
      exit : k = 0;
    state STOP
      entry: FA_START_ICE=0;
    STOP -> START : [(CMD_START_STOP ==0)]
    (default) -> STOP
    START -> STOP : [(CMD_START_STOP ==1)&&(k >200)]
  note: In the state START , we don't allowing a use of the ICE for less than 2 seconds
  (default) -> WAKEUP
  RUNNING -> WAKEUP : [(START == 0)]
  WAKEUP -> RUNNING : [(START == 1)]
  data: START input; CMD_START_STOP input; FA_START_ICE output; ENERGY_MANAGEMENT_ON_OFF output; k local
